simulink model "SiDrivetrain"  (R2017b)
settings: Solver=ode23tb  StartTime=0.0  StopTime=50  RelTol=1e-3  EnableMultiTasking=on
model workspace (MAT data in the model file):
  N = [-4.7 4.75 4.75 3.75 3.25 2.75 2.25 1.5 1 0.75]
  Ndiff = 3
  Re = 0.3
  MCOS : class17 (value not decoded)
  MCOS : class17 (value not decoded)
  MCOS : class17 (value not decoded)
  MCOS : class17 (value not decoded)
  MCOS : class17 (value not decoded)
  MCOS : class17 (value not decoded)
  MCOS : class17 (value not decoded)
  MCOS : class17 (value not decoded)
values from neighbouring files (symbols this model uses):
  b_axle = 10.0    [DrivetrainEvDD.sldd]    (also in DrivetrainHevMmDD.sldd; SiDrivetrainDD.sldd)
  b_driveshaft = 10.0    [DrivetrainEvDD.sldd]    (also in DrivetrainHevMmDD.sldd; SiDrivetrainDD.sldd)
  k_axle = 5000.0    [DrivetrainEvDD.sldd]    (also in DrivetrainHevMmDD.sldd; SiDrivetrainDD.sldd)
  k_driveshaft = 1000.0    [DrivetrainEvDD.sldd]    (also in DrivetrainHevMmDD.sldd; SiDrivetrainDD.sldd)
libraries: autolibsharedcoupling x12, autolibshared x7, autolibshareddiff x4, autolibutils x3, autolibcoupling x2, simulink x2, autolibsharedtransfixedgear x2, autolibtransdct x1, autolibshareddrivetraincommon x1, autolibtranscontrols x1
(part 5 of 5)

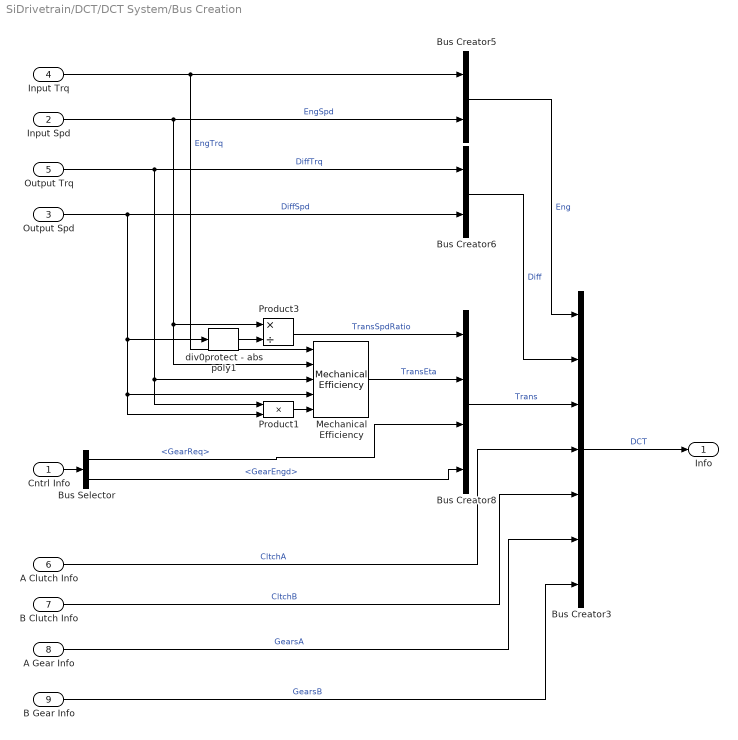
== system SiDrivetrain/DCT/DCT System/Bus Creation ==
  Cntrl Info : Inport
  Input Spd : Inport  Port=2  Unit=rad/s
  Output Spd : Inport  Port=3  Unit=rad/s
  Input Trq : Inport  Port=4  Unit=N*m
  Output Trq : Inport  Port=5  Unit=N*m
  A Clutch Info : Inport  Port=6
  B Clutch Info : Inport  Port=7
  A Gear Info : Inport  Port=8
  B Gear Info : Inport  Port=9
  Bus Creator3 : BusCreator  Inputs=7
  Bus Creator5 : BusCreator  Inputs=2
  Bus Creator6 : BusCreator  Inputs=2
  Bus Creator8 : BusCreator  Inputs=4
  Bus Selector : BusSelector  OutputSignals=GearReq,GearEngd
  Mechanical Efficiency : autolibshareddrivetraincommon/Mechanical Efficiency
      settings: SourceProductName=Powertrain Blockset  SourceProductBaseCode=PW
  Product1 : Product  Inputs=**
  Product3 : Product  Inputs=*/
  div0protect - abs poly1 : autolibutils/div0protect - abs poly  thresh=1e-6
      settings: SourceProductName=Powertrain Blockset  SourceProductBaseCode=PW
  Info : Outport
  wires:
  A Clutch Info/1 -> Bus Creator3/4  "CltchA"
  B Clutch Info/1 -> Bus Creator3/5  "CltchB"
  A Gear Info/1 -> Bus Creator3/6  "GearsA"
  B Gear Info/1 -> Bus Creator3/7  "GearsB"
  Bus Creator3/1 -> Info/1  "DCT"
  Bus Selector/1 -> Bus Creator8/3  "<GearReq>"
  Input Spd/1 -> Bus Creator5/2, Mechanical Efficiency/2, Product3/1  "EngSpd"
  Input Trq/1 -> Bus Creator5/1, Mechanical Efficiency/1  "EngTrq"
  Mechanical Efficiency/1 -> Bus Creator8/2  "TransEta"
  Output Spd/1 -> Bus Creator6/2, Product1/2, Mechanical Efficiency/4, div0protect - abs poly1/1  "DiffSpd"
  Output Trq/1 -> Bus Creator6/1, Product1/1, Mechanical Efficiency/3  "DiffTrq"
  Bus Selector/2 -> Bus Creator8/4  "<GearEngd>"
  Bus Creator8/1 -> Bus Creator3/3  "Trans"
  Product3/1 -> Bus Creator8/1  "TransSpdRatio"
  Product1/1 -> Mechanical Efficiency/5
  Bus Creator6/1 -> Bus Creator3/2  "Diff"
  Bus Creator5/1 -> Bus Creator3/1  "Eng"
  Cntrl Info/1 -> Bus Selector/1
  div0protect - abs poly1/1 -> Product3/2

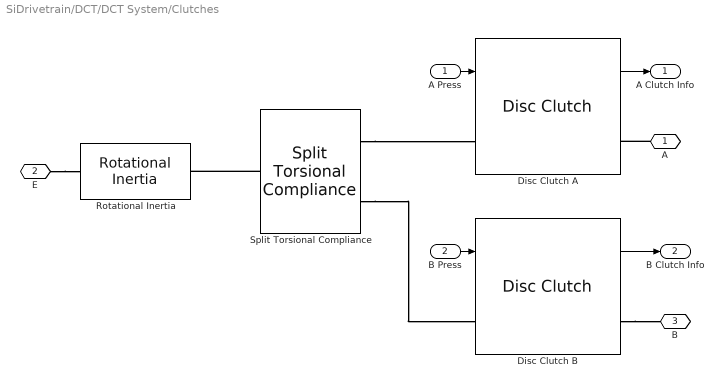
== system SiDrivetrain/DCT/DCT System/Clutches ==
  A Press : Inport
  B Press : Inport  Port=2
  Disc Clutch A : autolibcoupling/Disc Clutch  port_config=Two-way connection  Reff=.25  Ndisk=1  Aeff=.001  Jin=.05  Jout=.001  muk=.25  mus=.3  bin=.001  bout=.001  win_o=0  wout_o=0  tauC=.001  InitiallyLocked=off  maxAbsSpd=3000  blkID=1
      settings: SourceProductName=Powertrain Blockset  SourceProductBaseCode=PW
  Disc Clutch B : autolibcoupling/Disc Clutch  port_config=Two-way connection  Reff=.25  Ndisk=1  Aeff=.001  Jin=.05  Jout=.001  muk=.25  mus=.3  bin=.0001  bout=.0001  win_o=0  wout_o=0  tauC=.001  InitiallyLocked=off  maxAbsSpd=3000  blkID=1
      settings: SourceProductName=Powertrain Blockset  SourceProductBaseCode=PW
  Rotational Inertia : autolibsharedcoupling/Rotational Inertia  port_config=Two-way connection  J=.1  b=.001  omega_o=0  externJ=off  blkID=0
      settings: SourceProductName=Powertrain Blockset  SourceProductBaseCode=PW
  Split Torsional Compliance : autolibsharedcoupling/Split Torsional Compliance  port_config=Two-way connection  cplrMode=Shaft split  k1=5e3  b1=50  omega1_c=200  theta1_o=0  domega1_o=0  k2=5e3  b2=50  omega2_c=200  theta2_o=0  domega2_o=0  blkID=0
      settings: SourceProductName=Powertrain Blockset  SourceProductBaseCode=PW
  A : PMIOPort  Port=1  Side=Right
  E : PMIOPort  Port=2  Side=Left
  B : PMIOPort  Port=3  Side=Right
  A Clutch Info : Outport
  B Clutch Info : Outport  Port=2
  wires:
  Disc Clutch B/1 -> B Clutch Info/1
  B Press/1 -> Disc Clutch B/1
  A Press/1 -> Disc Clutch A/1
  Disc Clutch A/1 -> A Clutch Info/1
  connections:
  Split Torsional Compliance/RConn2 -- Disc Clutch B/LConn1
  E/RConn1 -- Rotational Inertia/LConn1
  Split Torsional Compliance/LConn1 -- Rotational Inertia/RConn1
  Split Torsional Compliance/RConn1 -- Disc Clutch A/LConn1
  A/RConn1 -- Disc Clutch A/RConn1
  Disc Clutch B/RConn1 -- B/RConn1

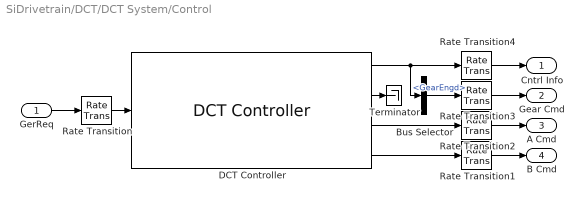
== system SiDrivetrain/DCT/DCT System/Control ==
  GerReq : Inport
  Bus Selector : BusSelector  OutputSignals=GearEngd
  DCT Controller : autolibtranscontrols/DCT Controller  G_o=0  tc=.5  ts=.01  dt=dt_DCT  ClutchLocked=off  SynchLocked=off
      settings: SourceProductName=Powertrain Blockset  SourceProductBaseCode=PW
  Rate Transition : RateTransition  Deterministic=off
  Rate Transition{1..4} (4 alike) : RateTransition
  Terminator : Terminator
  Cntrl Info : Outport
  Gear Cmd : Outport  Port=2
  A Cmd : Outport  Port=3
  B Cmd : Outport  Port=4
  wires:
  DCT Controller/1 -> Bus Selector/1, Rate Transition4/1
  Rate Transition/1 -> DCT Controller/1
  DCT Controller/3 -> Rate Transition2/1
  GerReq/1 -> Rate Transition/1
  DCT Controller/4 -> Rate Transition1/1
  DCT Controller/2 -> Terminator/1
  Rate Transition3/1 -> Gear Cmd/1
  Rate Transition4/1 -> Cntrl Info/1
  Rate Transition1/1 -> B Cmd/1
  Rate Transition2/1 -> A Cmd/1
  Bus Selector/1 -> Rate Transition3/1  "<GearEngd>"

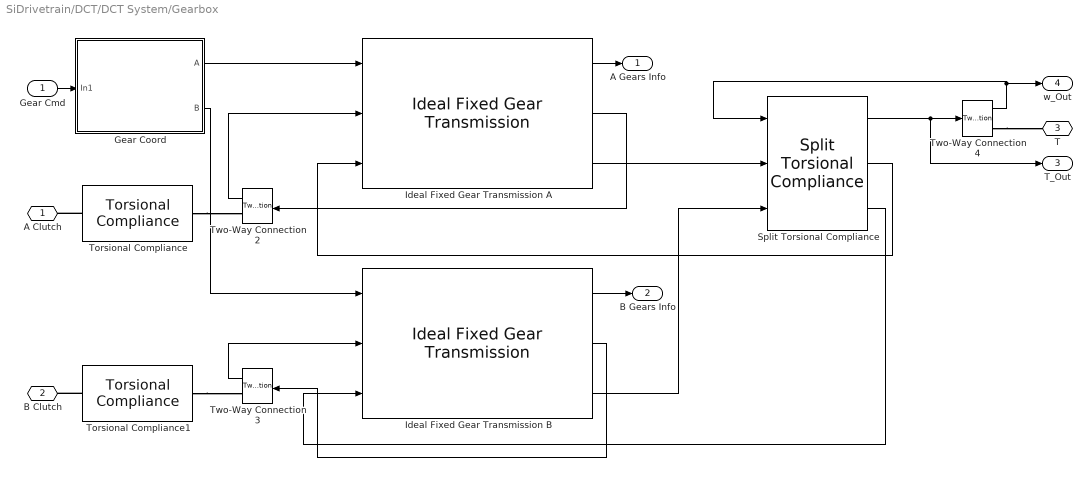
== system SiDrivetrain/DCT/DCT System/Gearbox ==
  Gear Cmd : Inport
  Gear Coord : Subsystem
  Ideal Fixed Gear Transmission A : autolibsharedtransfixedgear/Ideal Fixed Gear Transmission  VariantControl=0  G=[0,1,3,5,7]  N=[N(2), N(3:2:end)]  Jout=[0.28 0028 .2 0.11 0.11]  bout=[.001 .003 .002 .001 .001]  eta=[0.9, 0.9, 0.9, 0.9, 0.9]  omega_o=0  tau_s=.01  gearInterp=Nearest  maxAbsSpd=5e3
      settings: SourceProductName=Powertrain Blockset  SourceProductBaseCode=PW
  Ideal Fixed Gear Transmission B : autolibsharedtransfixedgear/Ideal Fixed Gear Transmission  VariantControl=0  G=[-1, 0, 2, 4, 6, 8]  N=[N(1), N(2:2:end)]  Jout="[0.28 0.24 0.24 0.18  0.11  0.11]"  bout=[0.003,0.001,0.0025,0.001,0.001,0.001]  eta=[0.9, 0.9, 0.9, 0.95, 0.95,0.95]  omega_o=0  tau_s=.01  gearInterp=Nearest  maxAbsSpd=5e3
      settings: SourceProductName=Powertrain Blockset  SourceProductBaseCode=PW
  Split Torsional Compliance : autolibsharedcoupling/Split Torsional Compliance  port_config=Simulink  cplrMode=Shaft merge  k1=5e3  b1=50  omega1_c=200  theta1_o=0  domega1_o=0  k2=5e3  b2=50  omega2_c=200  theta2_o=0  domega2_o=0  blkID=0
      settings: SourceProductName=Powertrain Blockset  SourceProductBaseCode=PW
  Torsional Compliance : autolibsharedcoupling/Torsional Compliance  port_config=Two-way connection  k=k_driveshaft  b=b_driveshaft  theta_o=0  domega_o=0  omega_c=wc_shaft  blkID=0
      settings: SourceProductName=Powertrain Blockset  SourceProductBaseCode=PW
  Torsional Compliance1 : autolibsharedcoupling/Torsional Compliance  port_config=Two-way connection  k=k_driveshaft  b=b_driveshaft  theta_o=0  domega_o=0  omega_c=wc_shaft  blkID=0
      settings: SourceProductName=Powertrain Blockset  SourceProductBaseCode=PW
  Two-Way Connection2 : TwoWayConnection
  Two-Way Connection3 : TwoWayConnection
  Two-Way Connection4 : TwoWayConnection
  A Clutch : PMIOPort  Port=1  Side=Left
  B Clutch : PMIOPort  Port=2  Side=Left
  T : PMIOPort  Port=3  Side=Right
  A Gears Info : Outport
  B Gears Info : Outport  Port=2
  T_Out : Outport  Port=3
  w_Out : Outport  Port=4
  wires:
  Ideal Fixed Gear Transmission B/1 -> B Gears Info/1
  Ideal Fixed Gear Transmission A/1 -> A Gears Info/1
  Ideal Fixed Gear Transmission B/2 -> Two-Way Connection3/1
  Gear Coord/2(B) -> Ideal Fixed Gear Transmission B/1
  Two-Way Connection2/1 -> Ideal Fixed Gear Transmission A/2
  Gear Cmd/1 -> Gear Coord/1(In1)
  Gear Coord/1(A) -> Ideal Fixed Gear Transmission A/1
  Two-Way Connection3/1 -> Ideal Fixed Gear Transmission B/2
  Ideal Fixed Gear Transmission A/2 -> Two-Way Connection2/1
  Ideal Fixed Gear Transmission B/3 -> Split Torsional Compliance/3
  Split Torsional Compliance/1 -> Two-Way Connection4/1, T_Out/1
  Two-Way Connection4/1 -> Split Torsional Compliance/1, w_Out/1
  Ideal Fixed Gear Transmission A/3 -> Split Torsional Compliance/2
  Split Torsional Compliance/3 -> Ideal Fixed Gear Transmission B/3
  Split Torsional Compliance/2 -> Ideal Fixed Gear Transmission A/3
  connections:
  Torsional Compliance1/LConn1 -- B Clutch/RConn1
  Torsional Compliance/RConn1 -- Two-Way Connection2/RConn1
  Torsional Compliance1/RConn1 -- Two-Way Connection3/RConn1
  Torsional Compliance/LConn1 -- A Clutch/RConn1
  Two-Way Connection4/RConn1 -- T/RConn1

== system SiDrivetrain/DCT/DCT System/Hydraulics ==
  Gear Cmd : Inport
  A Cmd : Inport  Port=2
  B Cmd : Inport  Port=3
  A Hydraulics Tau : Subsystem
  B Hydraulics Tau : Subsystem
  A Press : Outport
  B Press : Outport  Port=2
  wires:
  B Hydraulics Tau/1(Out1) -> B Press/1
  Gear Cmd/1 -> B Hydraulics Tau/1(In1), A Hydraulics Tau/1(In1)
  A Hydraulics Tau/1(Out1) -> A Press/1
  A Cmd/1 -> A Hydraulics Tau/2(In2)
  B Cmd/1 -> B Hydraulics Tau/2(In2)

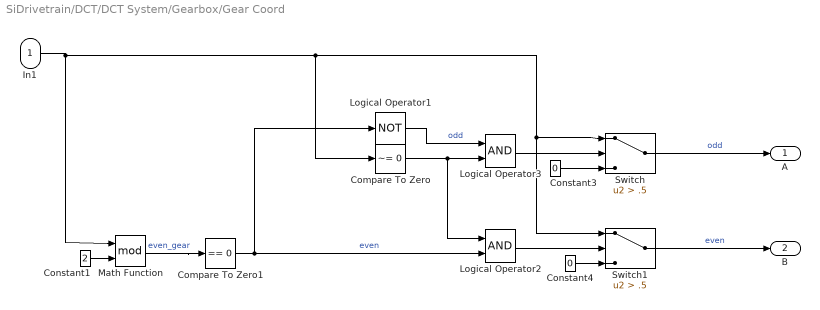
== system SiDrivetrain/DCT/DCT System/Gearbox/Gear Coord ==
  In1 : Inport
  Compare To Zero : simulink/Logic and Bit Operations/Compare To Zero  relop=~=  OutDataTypeStr=boolean
  Compare To Zero1 : simulink/Logic and Bit Operations/Compare To Zero  relop===  OutDataTypeStr=boolean
  Constant1 : Constant  Value=2
  Constant3 : Constant  Value=0
  Constant4 : Constant  Value=0
  Logical Operator1 : Logic  Operator=NOT  AllPortsSameDT=off  OutDataTypeStr=boolean
  Logical Operator2 : Logic  AllPortsSameDT=off  OutDataTypeStr=boolean
  Logical Operator3 : Logic  AllPortsSameDT=off  OutDataTypeStr=boolean
  Math Function : Math  Operator=mod  SaturateOnIntegerOverflow=on
  Switch : Switch  Criteria=u2 > Threshold  Threshold=.5
  Switch1 : Switch  Criteria=u2 > Threshold  Threshold=.5
  A : Outport
  B : Outport  Port=2
  wires:
  In1/1 -> Switch/1, Switch1/1, Compare To Zero/1, Math Function/1
  Math Function/1 -> Compare To Zero1/1  "even_gear"
  Constant1/1 -> Math Function/2
  Compare To Zero1/1 -> Logical Operator1/1, Logical Operator2/2  "even"
  Constant4/1 -> Switch1/3
  Switch/1 -> A/1  "odd"
  Constant3/1 -> Switch/3
  Switch1/1 -> B/1  "even"
  Logical Operator2/1 -> Switch1/2
  Logical Operator3/1 -> Switch/2
  Compare To Zero/1 -> Logical Operator2/1, Logical Operator3/2
  Logical Operator1/1 -> Logical Operator3/1  "odd"

== system SiDrivetrain/DCT/DCT System/Hydraulics/A Hydraulics Tau ==
  In1 : Inport
  In2 : Inport  Port=2
  2*pi : Gain  Gain=2*pi
  ClutchGain : Gain  Gain=k_hyd
  Constant1 : Constant  Value=0
  Constant2 : Constant  Value=tau_hyd
  Cont LPF Dyn : autolibutils/Cont LPF Dyn  SystemSampleTime=-1
      settings: SourceProductName=Powertrain Blockset  SourceProductBaseCode=PW
  Product : Product  Inputs=/
  Switch : Switch  Criteria=u2 ~= 0
  Out1 : Outport
  wires:
  In1/1 -> Switch/2
  ClutchGain/1 -> Out1/1
  Constant2/1 -> Product/1
  Cont LPF Dyn/1 -> ClutchGain/1
  Switch/1 -> Cont LPF Dyn/1
  Product/1 -> 2*pi/1
  In2/1 -> Switch/1
  2*pi/1 -> Cont LPF Dyn/2
  Constant1/1 -> Switch/3

== system SiDrivetrain/DCT/DCT System/Hydraulics/B Hydraulics Tau ==
  In1 : Inport
  In2 : Inport  Port=2
  2*pi : Gain  Gain=2*pi
  ClutchGain : Gain  Gain=k_hyd
  Constant1 : Constant  Value=0
  Constant2 : Constant  Value=tau_hyd
  Cont LPF Dyn : autolibutils/Cont LPF Dyn  SystemSampleTime=-1
      settings: SourceProductName=Powertrain Blockset  SourceProductBaseCode=PW
  Product : Product  Inputs=/
  Switch : Switch  Criteria=u2 ~= 0
  Out1 : Outport
  wires:
  Constant1/1 -> Switch/3
  2*pi/1 -> Cont LPF Dyn/2
  In2/1 -> Switch/1
  Product/1 -> 2*pi/1
  Switch/1 -> Cont LPF Dyn/1
  Cont LPF Dyn/1 -> ClutchGain/1
  Constant2/1 -> Product/1
  ClutchGain/1 -> Out1/1
  In1/1 -> Switch/2
